simulink model "MotorControl_HallSensor"  (R2014b)
settings: Solver=FixedStepDiscrete  StartTime=0.0  StopTime=10.0  FixedStep=1/5000  RelTol=1e-3
libraries: simulink x3, GPIO_Lib x2, ADC_Lib x1, STM32_Config_Lib x1, TIMERS_Lib x1
settings Model: SimulationMode=accelerator  Creator=Alex  LastModifiedBy=reynaudp
settings OptimizationCC: ExpressionDepthLimit=2147483647  OptimizeModelRefInitCode=on  LifeSpan=1
settings DebuggingCC: UnderspecifiedInitializationDetection=Classic  MergeDetectMultiDrivingBlocksExec=none  StateNameClashWarn=warning
settings HardwareCC: ProdLargestAtomicInteger=Integer  ProdLargestAtomicFloat=Float  ProdIntDivRoundTo=Zero  ProdEndianess=LittleEndian  ProdHWDeviceType=STMicroelectronics->STM32 32-bit Cortex-M  TargetLargestAtomicInteger=Integer  TargetLargestAtomicFloat=Float  TargetIntDivRoundTo=Zero  TargetEndianess=LittleEndian  TargetHWDeviceType=STMicroelectronics->STM32F4xx 32-bit Cortex-M4
settings RTWCC: SystemTargetFile=stm32.tlc  TemplateMakefile=stm32.tmf  Description=stm32 (Embedded Target)  GenerateReport=on  ProcessScript=stm32_make_rtw_hook  IncludeHyperlinkInReport=on
settings CodeAppCC: IgnoreCustomStorageClasses=off  MaxIdLength=64  CustomSymbolStrType=$N$R$M  SimulinkBlockComments=off  InternalIdentifier=Classic
settings STFCustomTargetCC: CodeReplacementLibrary=ARM CMSIS SIN COS  ParMdlRefBuildCompliant=on  IncludeMdlTerminateFcn=off  CombineOutputUpdateFcns=on  ERTCustomFileBanners=on  SupportContinuousTime=off  SupportNonInlinedSFcns=off  MATLABClassNameForMDSCustomization=Simulink.SoftwareTarget.ERTCustomization  GRTInterface=off  SystemTargetFile=stm32.tlc
settings ERTTargetCC: CodeReplacementLibrary=ARM CMSIS SIN COS  CompOptLevelCompliant=off  ConcurrentExecutionCompliant=off  IncludeMdlTerminateFcn=off  ERTFirstTimeCompliant=off  ModelStepFunctionPrototypeControlCompliant=off  CPPClassGenCompliant=off  InlinedParameterPlacement=NonHierarchical  ERTSrcFileBannerTemplate=sourceFileTemplate.cgt  ERTHdrFileBannerTemplate=sourceFileTemplate.cgt  ERTDataSrcFileTemplate=sourceFileTemplate.cgt  ERTDataHdrFileTemplate=sourceFileTemplate.cgt  ERTCustomFileTemplate=customRoutineProcess.tlc

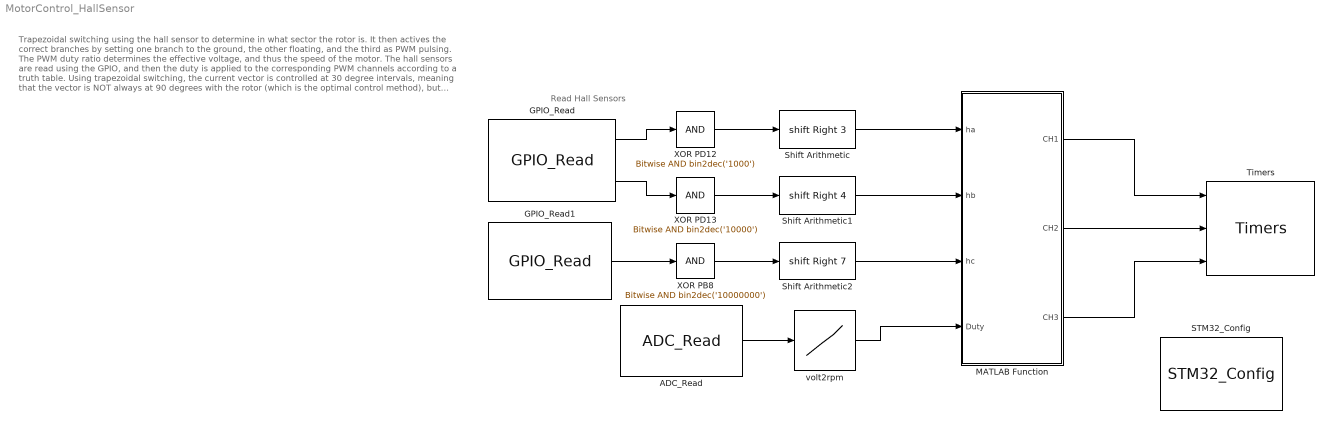
== system MotorControl_HallSensor ==
  note: Trapezoidal switching using the hall sensor to determine in what sector the rotor is. It then actives the correct branches by setting one branch to the ground, the other floating, and the third as PWM pulsing.
      |
      | The PWM duty ratio determines the effective voltage, and thus the speed of the motor. The hall sensors are read using the GPIO, and then the duty is applied to the corresponding PWM channels according to a truth table.
      |
      | Using trapezoidal switching, the current vector is controlled at 30 degree intervals, meaning that the vector is NOT always at 90 degrees with the rotor (which is the optimal control method), but rather oscillates with an error of +- 30 degrees. In this case, a ripple in the torque applied, and the motor produces extra noise, and consumes more current for the same mechanical power output (loss of efficiency)
      |
      | This Algorithm works in open loop (The motor speed is not measured)
  note: Read Hall Sensors
  ADC_Read : ADC_Lib/ADC_Read  ADC_Name=ADC3  ADC_Ch0=off  ADC_Ch1=off  ADC_Ch2=off  ADC_Ch3=off  ADC_Ch4=off  ADC_Ch5=off  ADC_Ch6=off  ADC_Ch7=on  ADC_Ch8=off  ADC_Ch9=off  ADC_Ch10=off  ADC_Ch11=off  ADC_Ch12=off  ADC_Ch13=off  ADC_Ch14=off  ADC_Ch15=off  ADC_Ch16=off  ADC_Ch17=off  ADC_Ch18=off  RgRk1=on  RgRk2=off  RgRk3=off  RgRk4=off  RgRk1_Ch=Ch7_r1  RgRk2_Ch=off  RgRk3_Ch=off  RgRk4_Ch=off  RgRk5=off  RgRk6=off  RgRk7=off  RgRk8=off  RgRk5_Ch=off  RgRk6_Ch=off  RgRk7_Ch=off  RgRk8_Ch=off  RgRk9=off  RgRk10=off  RgRk11=off  RgRk12=off  RgRk9_Ch=off  RgRk10_Ch=off  RgRk11_Ch=off  RgRk12_Ch=off  RgRk13=off  RgRk14=off  RgRk15=off  RgRk16=off  RgRk13_Ch=off  RgRk14_Ch=off  RgRk15_Ch=off  RgRk16_Ch=off  InjRk1=off  InjRk2=off  InjRk3=off  InjRk4=off  InjRk1_Ch=off  InjRk2_Ch=off  InjRk3_Ch=off  InjRk4_Ch=off  ADC_Trig=Not used  ADC_TrigEdge=Not used  DmaReq=off  ItReq=off  AWD_Mode=NOT_USED  AWD_Ch=0  AWD_HThres=0  AWD_LThres=0  AWD_En_Int=off  AWD2_HThres=0  AWD2_LThres=0  AWD2_En_Int=off  AWD3_HThres=0  AWD3_LThres=0  AWD3_En_Int=off  EOC_IT=off  JEOC_IT=off  AWD_IT=off  OVR_IT=off  ADC_RegNb=1  ADC_RegCh0=off  ADC_RegCh1=off  ADC_RegCh2=off  ADC_RegCh3=off  ADC_RegCh4=off  ADC_RegCh5=off  ADC_RegCh6=off  ADC_RegCh7=on  ADC_RegCh8=off  ADC_RegCh9=off  ADC_RegCh10=off  ADC_RegCh11=off  ADC_RegCh12=off  ADC_RegCh13=off  ADC_RegCh14=off  ADC_RegCh15=off  ADC_RegCh16=off  ADC_RegCh17=off  ADC_RegCh18=off  ADC_InjNb=0  ADC_InjCh0=off  ADC_InjCh1=off  ADC_InjCh2=off  ADC_InjCh3=off  ADC_InjCh4=off  ADC_InjCh5=off  ADC_InjCh6=off  ADC_InjCh7=off  ADC_InjCh8=off  ADC_InjCh9=off  ADC_InjCh10=off  ADC_InjCh11=off  ADC_InjCh12=off  ADC_InjCh13=off  ADC_InjCh14=off  ADC_InjCh15=off  ADC_InjCh16=off  ADC_InjCh17=off  ADC_InjCh18=off  ADC_RegRank0=0  ADC_RegRank1=0  ADC_RegRank2=0  ADC_RegRank3=0  ADC_RegRank4=0  ADC_RegRank5=0  ADC_RegRank6=0  ADC_RegRank7=1  ADC_RegRank8=0  ADC_RegRank9=0  ADC_RegRank10=0  ADC_RegRank11=0  ADC_RegRank12=0  ADC_RegRank13=0  ADC_RegRank14=0  ADC_RegRank15=0  ADC_RegRank16=0  ADC_RegRank17=0  ADC_RegRank18=0  ADC_InjRank0=0  ADC_InjRank1=0  ADC_InjRank2=0  ADC_InjRank3=0  ADC_InjRank4=0  ADC_InjRank5=0  ADC_InjRank6=0  ADC_InjRank7=0  ADC_InjRank8=0  ADC_InjRank9=0  ADC_InjRank10=0  ADC_InjRank11=0  ADC_InjRank12=0  ADC_InjRank13=0  ADC_InjRank14=0  ADC_InjRank15=0  ADC_InjRank16=0  ADC_InjRank17=0  ADC_InjRank18=0  NbADC=2  CurrentADC=ADC3
  GPIO_Read : GPIO_Lib/GPIO_Read  Port_name=GPIOD  Pin_0=off  Pin_1=off  Pin_2=off  Pin_3=off  Pin_4=off  Pin_5=off  Pin_6=off  Pin_7=off  Pin_8=off  Pin_9=off  Pin_10=off  Pin_11=off  Pin_12=on  Pin_13=on  Pin_14=off  Pin_15=off  PinList="GPIOB8GPIOD12  13"
  GPIO_Read1 : GPIO_Lib/GPIO_Read  Port_name=GPIOB  Pin_0=off  Pin_1=off  Pin_2=off  Pin_3=off  Pin_4=off  Pin_5=off  Pin_6=off  Pin_7=off  Pin_8=on  Pin_9=off  Pin_10=off  Pin_11=off  Pin_12=off  Pin_13=off  Pin_14=off  Pin_15=off  PinList="GPIOB8GPIOD12  13"
  MATLAB Function : MATLAB Function  TreatAsAtomicUnit=on
  STM32_Config : STM32_Config_Lib/STM32_Config  Priority=0  Project_Path=C:\snap_view\mcd_cd\Matlab\STM32\STM32demos\MotorControl\HallSensor\  Config_File=F407IGH6_Eval_HallSensor.ioc  MCU_Name=STM32F417IGHx
  Shift Arithmetic : ArithShift  BitShiftNumber=3  BitShiftDirection=Right
  Shift Arithmetic1 : ArithShift  BitShiftNumber=4  BitShiftDirection=Right
  Shift Arithmetic2 : ArithShift  BitShiftNumber=7  BitShiftDirection=Right
  Timers : TIMERS_Lib/Timers  currentTIM=TIM8  TIM_Name=TIM8  TIM_APBClock=168000000  TIM_CKD=1  TIM_Set_Clk=on  TIM_Prescaler=7  TIM_Clock=21000000.00  Variable_frequency=off  TIM_Set_OutFreq=on  TIM_ARR=525  Output_frequency=40000.00  Repetition_counter=0  TIM_Mode=Center_Aligned_2  TIM_DMA=none  TIM_IRQ=off  TIM_IRQ_ONLY=off  TIM_UP=off  TIM_TRG=off  TIM_COM=off  TIM_BRK=off  NbTIM=1  CH1_enable=on  CH1N_enable=on  CH1_type=Output_PWM  CH1_DMA=off  CH1_int=off  CH1_edge=Rising  CH1_div=1  CH1_variable_duty=on  CH1_set_pulse=on  CH1_output_duty=50  CH1_pulse=262  CH2_enable=on  CH2N_enable=on  CH2_type=Output_PWM  CH2_DMA=off  CH2_int=off  CH2_edge=Rising  CH2_div=1  CH2_variable_duty=on  CH2_set_pulse=on  CH2_output_duty=50  CH2_pulse=262  CH3_enable=on  CH3N_enable=on  CH3_type=Output_PWM  CH3_DMA=off  CH3_int=off  CH3_edge=Rising  CH3_div=1  CH3_variable_duty=on  CH3_set_pulse=on  CH3_output_duty=50  CH3_pulse=262  CH4_enable=off  CH4N_enable=off  CH4_type=Unknown  CH4_DMA=off  CH4_int=off  CH4_edge=Rising  CH4_div=1  CH4_variable_duty=off  CH4_set_pulse=off  CH4_output_duty=0.00  CH4_pulse=0
  XOR PB8 : simulink/Logic and Bit Operations/Bitwise Operator  logicop=AND  UseBitMask=on  BitMask=bin2dec('10000000')  BitMaskRealWorld=Stored Integer
  XOR PD12 : simulink/Logic and Bit Operations/Bitwise Operator  logicop=AND  UseBitMask=on  BitMask=bin2dec('1000')  BitMaskRealWorld=Stored Integer
  XOR PD13 : simulink/Logic and Bit Operations/Bitwise Operator  logicop=AND  UseBitMask=on  BitMask=bin2dec('10000')  BitMaskRealWorld=Stored Integer
  volt2rpm : Lookup_n-D  NumberOfTableDimensions=1  BreakpointsForDimension1=[0:100]*(4095/100)  BreakpointsForDimension1Min=0  BreakpointsForDimension1Max=4095  Table=[0:100]  RndMeth=Simplest  InputSameDT=on
  wires:
  XOR PD12/1 -> Shift Arithmetic/1
  XOR PD13/1 -> Shift Arithmetic1/1
  XOR PB8/1 -> Shift Arithmetic2/1
  MATLAB Function/2(CH2) -> Timers/2
  MATLAB Function/1(CH1) -> Timers/1
  MATLAB Function/3(CH3) -> Timers/3
  Shift Arithmetic1/1 -> MATLAB Function/2(hb)
  volt2rpm/1 -> MATLAB Function/4(Duty)
  Shift Arithmetic/1 -> MATLAB Function/1(ha)
  Shift Arithmetic2/1 -> MATLAB Function/3(hc)
  GPIO_Read1/1 -> XOR PB8/1
  GPIO_Read/1 -> XOR PD12/1
  GPIO_Read/2 -> XOR PD13/1
  ADC_Read/1 -> volt2rpm/1

== matlab function MotorControl_HallSensor/MATLAB Function ==
  data: ha input; hb input; hc input; CH1 output; CH2 output; CH3 output; Duty input
function [CH1,CH2,CH3]=Hall_State(ha,hb,hc,Duty)

bc = ha & hb & ~hc;
ba = ~ha & hb & ~hc;
ca = ~ha & hb & hc;
cb = ~ha & ~hb & hc;
ab = ha & ~hb & hc;
ac = ha & ~hb & ~hc;

if bc
    CH1 = (-1);
    CH2 = (Duty);
    CH3 = (0);
elseif ba
    CH1 = (0);
    CH2 = (Duty);
    CH3 = (-1);
elseif ca
    CH1 = (0);
    CH2 = (-1);
    CH3 = (Duty);
elseif cb
    CH1 = (-1);
    CH2 = (0);
    CH3 = (Duty);
elseif ab
    CH1 = (Duty);
    CH2 = (0);
    CH3 = (-1);
elseif ac
    CH1 = (Duty);
    CH2 = (-1);
    CH3 = (0);
else
    CH1 = (-1);
    CH2 = (-1);
    CH3 = (-1);
end
